simulink model "Reductor"  (R2023a)
settings: Solver=VariableStepAuto  StartTime=0.0  StopTime=1  RelTol=1e-3
undefined symbols (not defined in the file): a, c, F1, F2, G, G1, G2, i, J
settings Model: Creator=manui  LastModifiedBy=manui

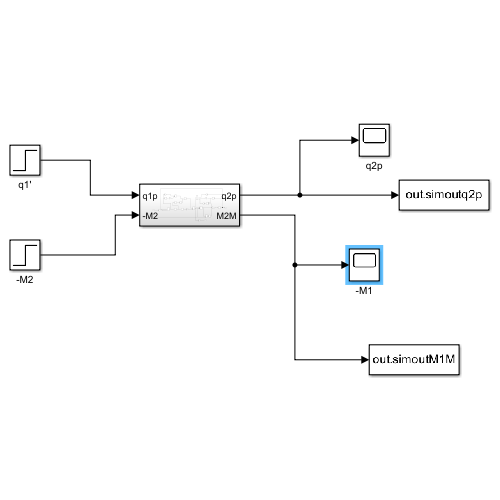
[thumbnail: Simulink's stored preview of the top-level diagram]
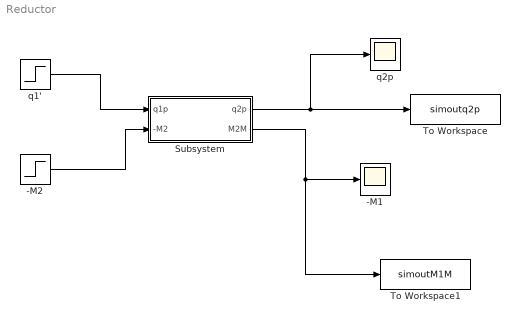
== system Reductor ==
  -M1 : Scope
  -M2 : Step  Time=0  SampleTime=0
  Subsystem : Subsystem
  To Workspace : ToWorkspace  VariableName=simoutq2p  SaveFormat=Timeseries  SampleTime=-1
  To Workspace1 : ToWorkspace  VariableName=simoutM1M  SaveFormat=Timeseries  SampleTime=-1
  q1' : Step  Time=0  SampleTime=0
  q2p : Scope
  wires:
  q1'/1 -> Subsystem/1(q1p)
  -M2/1 -> Subsystem/2(-M2)
  Subsystem/1(q2p) -> To Workspace/1, q2p/1
  Subsystem/2(M2M) -> To Workspace1/1, -M1/1

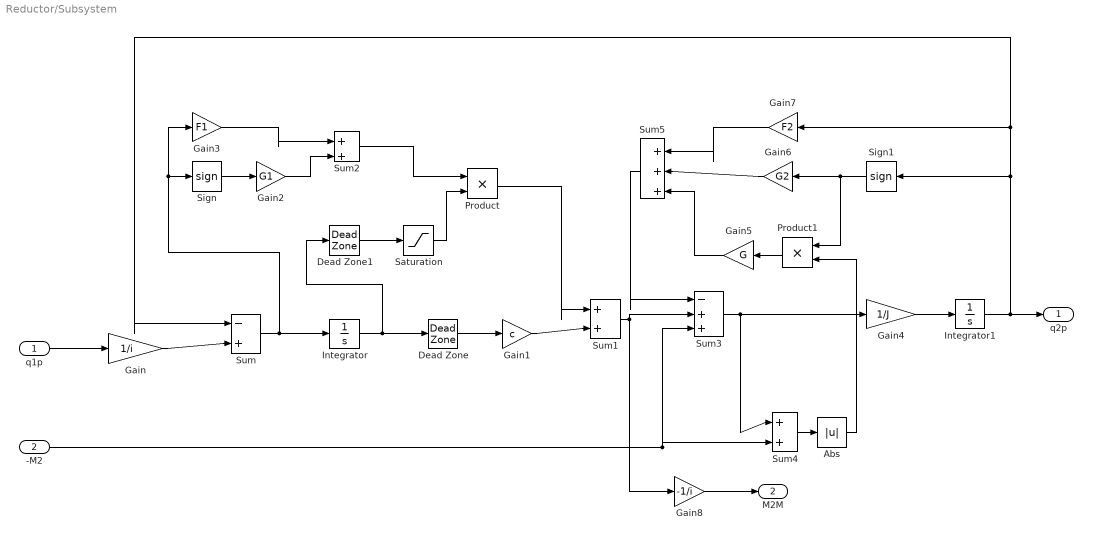
== system Reductor/Subsystem ==
  q1p : Inport
  -M2 : Inport  Port=2
  Abs : Abs  SaturateOnIntegerOverflow=off
  Dead Zone : DeadZone  LowerValue=-a  UpperValue=a
  Dead Zone1 : DeadZone  LowerValue=-a  UpperValue=a
  Gain : Gain  Gain=1/i
  Gain1 : Gain  Gain=c
  Gain2 : Gain  Gain=G1
  Gain3 : Gain  Gain=F1
  Gain4 : Gain  Gain=1/J
  Gain5 : Gain  Gain=G
  Gain6 : Gain  Gain=G2
  Gain7 : Gain  Gain=F2
  Gain8 : Gain  Gain=-1/i
  Integrator : Integrator
  Integrator1 : Integrator
  Product : Product
  Product1 : Product
  Saturation : Saturate  UpperLimit=a  LowerLimit=-a
  Sign : Signum
  Sign1 : Signum
  Sum : Sum  Inputs=|-+
  Sum1 : Sum  Inputs=|++
  Sum2 : Sum  Inputs=|++
  Sum3 : Sum  Inputs=|-++
  Sum4 : Sum  Inputs=|++
  Sum5 : Sum  Inputs=|+++
  q2p : Outport
  M2M : Outport  Port=2
  wires:
  q1p/1 -> Gain/1
  Gain/1 -> Sum/2
  Sum/1 -> Sign/1, Gain3/1, Integrator/1
  Integrator/1 -> Dead Zone1/1, Dead Zone/1
  Dead Zone/1 -> Gain1/1
  Gain1/1 -> Sum1/2
  Product/1 -> Sum1/1
  Saturation/1 -> Product/2
  Dead Zone1/1 -> Saturation/1
  Gain2/1 -> Sum2/2
  Sum2/1 -> Product/1
  Gain3/1 -> Sum2/1
  Sign/1 -> Gain2/1
  Sum1/1 -> Gain8/1, Sum3/2
  -M2/1 -> Sum3/3, Sum4/2
  Gain4/1 -> Integrator1/1
  Integrator1/1 -> Sum/1, Gain7/1, Sign1/1, q2p/1
  Sum3/1 -> Sum4/1, Gain4/1
  Sum4/1 -> Abs/1
  Abs/1 -> Product1/2
  Product1/1 -> Gain5/1
  Gain5/1 -> Sum5/3
  Gain6/1 -> Sum5/2
  Sign1/1 -> Product1/1, Gain6/1
  Gain7/1 -> Sum5/1
  Gain8/1 -> M2M/1
  Sum5/1 -> Sum3/1
